simulink model "NOTTest"  (R2016a)
settings: Solver=VariableStepAuto  StartTime=0.0  StopTime=1  RelTol=1e-3
libraries: SimscapeMacros x4, ProjectBlocks x1, nesl_utility x1
settings Model: Creator=Peter  LastModifiedBy=Peter

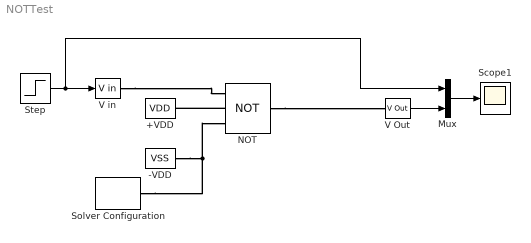
== system NOTTest ==
  +VDD : SimscapeMacros/VDD
  -VDD : SimscapeMacros/VSS
  Mux : Mux  Inputs=2
  NOT : ProjectBlocks/NOT
  Scope1 : Scope
  Solver Configuration : nesl_utility/Solver Configuration  PhysicalDomain=network_engine_domain  SubClassName=solver  LeftPortType=input  RightPortType=generic  Accelerate=off  Tones=[]  Harmonics=[]  SimulateNoise=off  Profile=off  UseLocalSampling=off  EnableSwitchedLinearOptims=on  FrequencyDomain=off  UseCCode=off  RelTol=0.001  AbsTol=1e-06  MinStep=1e-09  ToWorkspace=off  RevertToSquareIcSolve=off  NumHomotopyIterations=100  PhasorMode=off  PhasorModeNumHarmonics=1  OverrideAbsTol=off  DoDC=off  ResidualTolerance=1e-09  UseLocalSolver=off  LocalSolverChoice=NE_BACKWARD_EULER_ADVANCER  LocalSolverSampleTime=0.001  DoFixedCost=off  MaxNonlinIter=3  MaxModeIter=2  LinearAlgebra=Sparse  DelaysMemoryBudget=1024  AutomaticFiltering=on  FilteringTimeConstant=0.001
  Step : Step  Time=.5  Before=-10  After=10  SampleTime=0
  V Out : SimscapeMacros/V Out
  V in : SimscapeMacros/V in
  wires:
  Step/1 -> V in/1, Mux/1
  Mux/1 -> Scope1/1
  V Out/1 -> Mux/2
  connections:
  V in/RConn1 -- NOT/LConn1
  NOT/RConn1 -- V Out/LConn1
  NOT/LConn2 -- +VDD/RConn1
  Solver Configuration/RConn1 -- NOT/LConn3 -- -VDD/RConn1
